simulink model "motor_kit_sim_20MHz"  (R2021b)
settings: Solver=VariableStepAuto  StartTime=0.0  StopTime=10*62.5E-6  RelTol=1e-3  EnableMultiTasking=on
PreLoadFcn:
  | setup_motor_kit_sim_20MHz;
InitFcn:
  | setup_motor_kit_sim_20MHz;
values from neighbouring files (symbols this model uses):
  DSPBASampleTime = 0.05e-6    (= 5e-08)    [setup_motor_kit_sim_20MHz.m]
  wordLength = 16    [setup_motor_kit_sim_20MHz.m]
undefined symbols (not defined in the file or in its folder): AdvDSPBChannelOutDisplay, dpoly, dspba_ChannelInVis, dspba_ChannelOutVis, dspba_internal_get_channel_ports, evalAionMaskParam, latency, primtype, value, x
libraries: DSPBAPrim x324, DSPBAModelBus x25, DSPBABase x7, dspsrcs4 x3, simulink x3, DSPBAUtilities x1
(part 4 of 5)

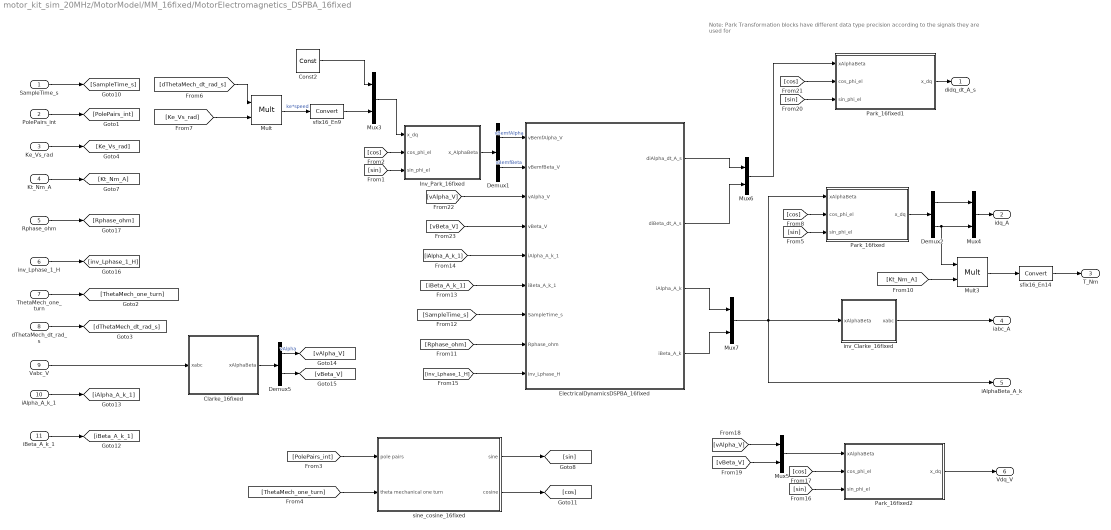
== system motor_kit_sim_20MHz/MotorModel/MM_16fixed/MotorElectromagnetics_DSPBA_16fixed ==
  note: Note: Park Transformation blocks have different data type precision according to the signals they are used for
  SampleTime_s : Inport
  PolePairs_int : Inport  Port=2
  Ke_Vs_rad : Inport  Port=3
  Kt_Nm_A : Inport  Port=4
  Rphase_ohm : Inport  Port=5
  inv_Lphase_1_H : Inport  Port=6
  ThetaMech_one_turn : Inport  Port=7
  dThetaMech_dt_rad_s : Inport  Port=8
  Vabc_V : Inport  Port=9
  iAlpha_A_k_1 : Inport  Port=10
  iBeta_A_k_1 : Inport  Port=11
  Clarke_16fixed : Subsystem
  Const2 : DSPBAPrim/Const  primtype=const  nInputs=0  nOutputs=1  omode=Specify via dialog  otype=DataType  scale=constScaleVoltage  rndmethod=Unbiased  factor=1  satmethod=Symmetric  shift_vec=[0 1 2 -1]  value=0  inPortNames=['+'; '+';]  outPortNames=[' ']  dspbaimage=dspba_prim.svg  text=fprintf('%s', num2str(value));  style=Optimised  visibilities=8 + 1024  floatPrecision=float32_m23  warnSaturation=on  version=20211007  SampleTime=inf
  Demux1 : Demux  Outputs=2
  Demux2 : Demux  Outputs=2
  Demux5 : Demux  Outputs=2
  ElectricalDynamicsDSPBA_16fixed : Subsystem
  Inv_Park_16fixed : Subsystem
  Mult : DSPBAPrim/Mult  primtype=mult  nInputs=2  nOutputs=1  omode=Inherit via internal rule  otype=DataType  scale=constScaleVoltage  rndmethod=Unbiased  factor=1  satmethod=Symmetric  shift_vec=[0 1 2 -1]  value=0  inPortNames=[' '; ' ';]  outPortNames=[' ']  dspbaimage=dspba_prim.svg  text=fprintf('X');  style=Optimised  visibilities=8+2^18+2^19  floatPrecision=float32_m23  floatRounding=correct  advOptions=[]  version=20211007
  Mult3 : DSPBAPrim/Mult  primtype=mult  nInputs=2  nOutputs=1  omode=Inherit via internal rule  otype=DataType  scale=constScaleTorque  rndmethod=Unbiased  factor=1  satmethod=Symmetric  shift_vec=[0 1 2 -1]  value=0  inPortNames=[' '; ' ';]  outPortNames=[' ']  dspbaimage=dspba_prim.svg  text=fprintf('X');  style=Optimised  visibilities=8+2^18+2^19  floatPrecision=float32_m23  floatRounding=correct  advOptions=[]  version=20211007
  Mux{3..7} (5 alike) : Mux  Inputs=2
  Park_16fixed : Subsystem
  Park_16fixed1 : Subsystem
  Park_16fixed2 : Subsystem
  inv_Clarke_16fixed : Subsystem
  sfix16_En14 : DSPBAPrim/Convert  primtype=convert  nInputs=1  nOutputs=1  omode=Specify via dialog  otype=DataTypeTorque  scale=constScaleTorque  rndmethod=Unbiased  factor=1  satmethod=Symmetric  shift_vec=[0 1 2 -1]  value=round([0:255]/17)  inPortNames=[' '; ' ';]  outPortNames=[' '; 'c']  dspbaimage=dspba_prim_wide.svg  text=fprintf('convert');  style=Optimised  visibilities=8+64+256+2^17  clipdetect=off  floatPrecision=float32_m23  advOptions=[]  version=20211007
  sfix16_En9 : DSPBAPrim/Convert  primtype=convert  nInputs=1  nOutputs=1  omode=Specify via dialog  otype=DataType  scale=constScaleVoltage  rndmethod=Unbiased  factor=1  satmethod=Symmetric  shift_vec=[0 1 2 -1]  value=round([0:255]/17)  inPortNames=[' '; ' ';]  outPortNames=[' '; 'c']  dspbaimage=dspba_prim_wide.svg  text=fprintf('convert');  style=Optimised  visibilities=8+64+256+2^17  clipdetect=off  floatPrecision=float32_m23  advOptions=[]  version=20211007
  sine_cosine_16fixed : Subsystem
  didq_dt_A_s : Outport
  idq_A : Outport  Port=2
  T_Nm : Outport  Port=3
  iabc_A : Outport  Port=4
  iAlphaBeta_A_k : Outport  Port=5
  Vdq_V : Outport  Port=6
  wires:
  Mult3/1 -> sfix16_En14/1
  [Kt_Nm_A] -> Mult3/2
  sine_cosine_16fixed/2(cosine) -> [cos]
  sine_cosine_16fixed/1(sine) -> [sin]
  [ThetaMech_one_turn] -> sine_cosine_16fixed/2(theta mechanical one turn)
  [PolePairs_int] -> sine_cosine_16fixed/1(pole pairs)
  Park_16fixed2/1(x_dq) -> Vdq_V/1
  [sin] -> Park_16fixed2/3(sin_phi_el)
  [cos] -> Park_16fixed2/2(cos_phi_el)
  Mux5/1 -> Park_16fixed2/1(xAlphaBeta)
  [vAlpha_V] -> Mux5/1
  [vBeta_V] -> Mux5/2
  inv_Clarke_16fixed/1(xabc) -> iabc_A/1
  Mux7/1 -> iAlphaBeta_A_k/1, Park_16fixed/1(xAlphaBeta), inv_Clarke_16fixed/1(xAlphaBeta)
  Mux4/1 -> idq_A/1
  Demux2/2 -> Mux4/2, Mult3/1
  Demux2/1 -> Mux4/1
  [sin] -> Park_16fixed/3(sin_phi_el)
  [cos] -> Park_16fixed/2(cos_phi_el)
  Park_16fixed/1(x_dq) -> Demux2/1
  Park_16fixed1/1(x_dq) -> didq_dt_A_s/1
  ElectricalDynamicsDSPBA_16fixed/2(diBeta_dt_A_s) -> Mux6/2
  ElectricalDynamicsDSPBA_16fixed/1(diAlpha_dt_A_s) -> Mux6/1
  [sin] -> Inv_Park_16fixed/3(sin_phi_el)
  [cos] -> Inv_Park_16fixed/2(cos_phi_el)
  [cos] -> Park_16fixed1/2(cos_phi_el)
  Mux6/1 -> Park_16fixed1/1(xAlphaBeta)
  [sin] -> Park_16fixed1/3(sin_phi_el)
  [inv_Lphase_1_H] -> ElectricalDynamicsDSPBA_16fixed/9(inv_Lphase_H)
  [Rphase_ohm] -> ElectricalDynamicsDSPBA_16fixed/8(Rphase_ohm)
  [SampleTime_s] -> ElectricalDynamicsDSPBA_16fixed/7(SampleTime_s)
  [iBeta_A_k_1] -> ElectricalDynamicsDSPBA_16fixed/6(iBeta_A_k_1)
  [iAlpha_A_k_1] -> ElectricalDynamicsDSPBA_16fixed/5(iAlpha_A_k_1)
  Mult/1 -> sfix16_En9/1  "ke*speed"
  [Ke_Vs_rad] -> Mult/2
  [dThetaMech_dt_rad_s] -> Mult/1
  Const2/1 -> Mux3/1
  iBeta_A_k_1/1 -> [iBeta_A_k_1]
  iAlpha_A_k_1/1 -> [iAlpha_A_k_1]
  dThetaMech_dt_rad_s/1 -> [dThetaMech_dt_rad_s]
  ThetaMech_one_turn/1 -> [ThetaMech_one_turn]
  inv_Lphase_1_H/1 -> [inv_Lphase_1_H]
  Rphase_ohm/1 -> [Rphase_ohm]
  Kt_Nm_A/1 -> [Kt_Nm_A]
  Ke_Vs_rad/1 -> [Ke_Vs_rad]
  SampleTime_s/1 -> [SampleTime_s]
  PolePairs_int/1 -> [PolePairs_int]
  Mux3/1 -> Inv_Park_16fixed/1(x_dq)
  Demux1/2 -> ElectricalDynamicsDSPBA_16fixed/2(vBemfBeta_V)  "vBemfBeta"
  Demux1/1 -> ElectricalDynamicsDSPBA_16fixed/1(vBemfAlpha_V)  "vBemfAlpha"
  Inv_Park_16fixed/1(x_AlphaBeta) -> Demux1/1
  [vAlpha_V] -> ElectricalDynamicsDSPBA_16fixed/3(vAlpha_V)
  [vBeta_V] -> ElectricalDynamicsDSPBA_16fixed/4(vBeta_V)
  Clarke_16fixed/1(xAlphaBeta) -> Demux5/1
  Demux5/2 -> [vBeta_V]
  Demux5/1 -> [vAlpha_V]  "vAlpha"
  Vabc_V/1 -> Clarke_16fixed/1(xabc)
  sfix16_En9/1 -> Mux3/2
  ElectricalDynamicsDSPBA_16fixed/4(iBeta_A_k) -> Mux7/2
  ElectricalDynamicsDSPBA_16fixed/3(iAlpha_A_k) -> Mux7/1
  sfix16_En14/1 -> T_Nm/1

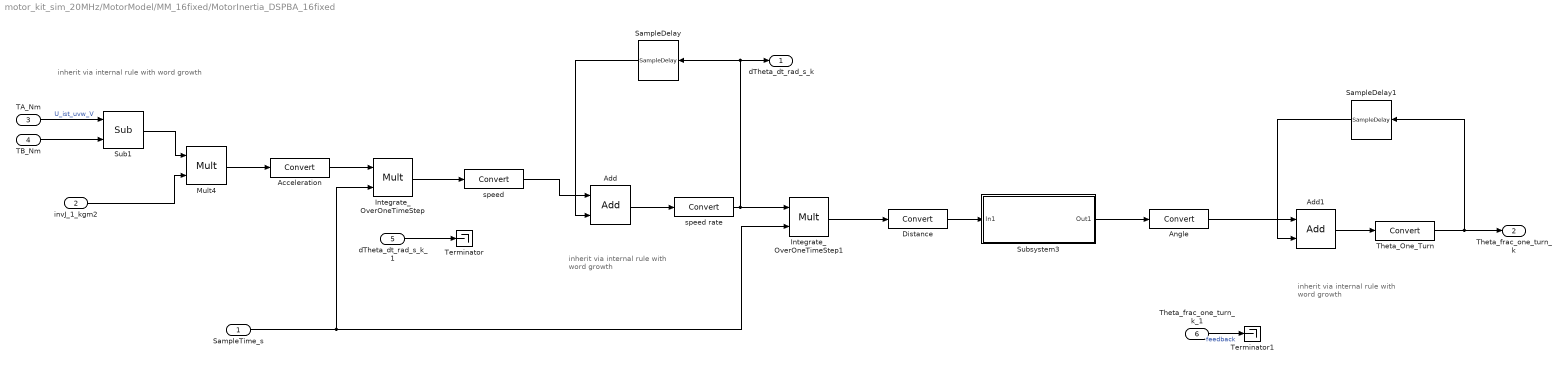
== system motor_kit_sim_20MHz/MotorModel/MM_16fixed/MotorInertia_DSPBA_16fixed ==
  note: inherit via internal rule with word growth
  note: inherit via internal rule
      | with word growth
  note: inherit via internal rule
      | with word growth
  SampleTime_s : Inport
  invJ_1_kgm2 : Inport  Port=2
  TA_Nm : Inport  Port=3
  TB_Nm : Inport  Port=4
  dTheta_dt_rad_s_k_1 : Inport  Port=5
  Theta_frac_one_turn_k_1 : Inport  Port=6
  Acceleration : DSPBAPrim/Convert  primtype=convert  nInputs=1  nOutputs=1  omode=Specify via dialog  otype=DataTypeAcceleration  scale=constScaleAcceleration  rndmethod=Truncate  factor=1  satmethod=None  shift_vec=[0 1 2 -1]  value=round([0:255]/17)  inPortNames=[' '; ' ';]  outPortNames=[' '; 'c']  dspbaimage=dspba_prim_wide.svg  text=fprintf('convert');  style=Optimised  visibilities=8+64+256+2^17  clipdetect=off  floatPrecision=float32_m23  advOptions=[]  version=20211007
  Add : DSPBAPrim/Add  primtype=add  nInputs=evalAionMaskParam(gcb,'value',1)  nOutputs=1  omode=Inherit via internal rule with word growth  otype=DataType  scale=constScaleSpeed  rndmethod=Unbiased  factor=1  satmethod=Symmetric  shift_vec=[0 1 2 -1]  value=2  inPortNames=[' '; ' ';]  outPortNames=[' ']  dspbaimage=dspba_prim.svg  text=fprintf('+');  style=Optimised  visibilities=1032  genFPC=off  floatRounding=correct  advOptions=[]  version=20211007
  Add1 : DSPBAPrim/Add  primtype=add  nInputs=evalAionMaskParam(gcb,'value',1)  nOutputs=1  omode=Inherit via internal rule with word growth  otype=DataTypeUnsigned  scale=2^-16  rndmethod=Unbiased  factor=1  satmethod=Symmetric  shift_vec=[0 1 2 -1]  value=2  inPortNames=[' '; ' ';]  outPortNames=[' ']  dspbaimage=dspba_prim.svg  text=fprintf('+');  style=Optimised  visibilities=1032  genFPC=off  floatRounding=correct  advOptions=[]  version=20211007
  Angle : DSPBAPrim/Convert  primtype=convert  nInputs=1  nOutputs=1  omode=Specify via dialog  otype=DataTypeTheta_OneTurn  scale=constScaleTheta_OneTurn  rndmethod=Unbiased  factor=1  satmethod=None  shift_vec=[0 1 2 -1]  value=round([0:255]/17)  inPortNames=[' '; ' ';]  outPortNames=[' '; 'c']  dspbaimage=dspba_prim_wide.svg  text=fprintf('convert');  style=Optimised  visibilities=8+64+256+2^17  clipdetect=off  floatPrecision=float32_m23  advOptions=[]  version=20211007
  Distance : DSPBAPrim/Convert  primtype=convert  nInputs=1  nOutputs=1  omode=Specify via dialog  otype=DataTypeDis  scale=constScaleDis  rndmethod=Unbiased  factor=1  satmethod=None  shift_vec=[0 1 2 -1]  value=round([0:255]/17)  inPortNames=[' '; ' ';]  outPortNames=[' '; 'c']  dspbaimage=dspba_prim_wide.svg  text=fprintf('convert');  style=Optimised  visibilities=8+64+256+2^17  clipdetect=off  floatPrecision=float32_m23  advOptions=[]  version=20211007
  Integrate_OverOneTimeStep : DSPBAPrim/Mult  primtype=mult  nInputs=2  nOutputs=1  omode=Inherit via internal rule  otype=DataType  scale=2^-12  rndmethod=Unbiased  factor=1  satmethod=Symmetric  shift_vec=[0 1 2 -1]  value=0  inPortNames=[' '; ' ';]  outPortNames=[' ']  dspbaimage=dspba_prim.svg  text=fprintf('X');  style=Optimised  visibilities=8+2^18+2^19  floatPrecision=float32_m23  floatRounding=correct  advOptions=[]  version=20211007
  Integrate_OverOneTimeStep1 : DSPBAPrim/Mult  primtype=mult  nInputs=2  nOutputs=1  omode=Inherit via internal rule  otype=sfix(32)  scale=2^-28  rndmethod=Unbiased  factor=1  satmethod=Symmetric  shift_vec=[0 1 2 -1]  value=0  inPortNames=[' '; ' ';]  outPortNames=[' ']  dspbaimage=dspba_prim.svg  text=fprintf('X');  style=Optimised  visibilities=8+2^18+2^19  floatPrecision=float32_m23  floatRounding=correct  advOptions=[]  version=20211007
  Mult4 : DSPBAPrim/Mult  primtype=mult  nInputs=2  nOutputs=1  omode=Inherit via internal rule  otype=DataTypeAcceleration  scale=2^0  rndmethod=Unbiased  factor=1  satmethod=Symmetric  shift_vec=[0 1 2 -1]  value=0  inPortNames=[' '; ' ';]  outPortNames=[' ']  dspbaimage=dspba_prim.svg  text=fprintf('X');  style=Optimised  visibilities=8+2^18+2^19  floatPrecision=float32_m23  floatRounding=correct  advOptions=[]  version=20211007
  SampleDelay : DSPBAPrim/SampleDelay  primtype=sampdelay  nInputs=1  nOutputs=1  omode=Inherit via internal rule  otype=sfix(16)  scale=2^-15  rndmethod=Unbiased  factor=1  satmethod=Symmetric  shift_vec=[0 1 2 -1]  floatPrecision=float32_m23  value=1  inPortNames=[' '; ' ';]  outPortNames=[' ']  dspbaimage=dspba_prim.svg  text=dpoly(1, eye(1,value+1), 'z')  style=Optimised  visibilities=8 + 1024 + 2^17 + 2^18  flexible=off  slackgroup=0  augmented=0  version=20211007  advOptions=[]
  SampleDelay1 : DSPBAPrim/SampleDelay  primtype=sampdelay  nInputs=1  nOutputs=1  omode=Inherit via internal rule  otype=sfix(16)  scale=2^-15  rndmethod=Unbiased  factor=1  satmethod=Symmetric  shift_vec=[0 1 2 -1]  floatPrecision=float32_m23  value=1  inPortNames=[' '; ' ';]  outPortNames=[' ']  dspbaimage=dspba_prim.svg  text=dpoly(1, eye(1,value+1), 'z')  style=Optimised  visibilities=8 + 1024 + 2^17 + 2^18  flexible=off  slackgroup=0  augmented=0  version=20211007  advOptions=[]
  Sub1 : DSPBAPrim/Sub  primtype=sub  nInputs=2  nOutputs=1  omode=Inherit via internal rule with word growth  otype=DataType  scale=constScaleTorque  rndmethod=Unbiased  factor=1  satmethod=Symmetric  shift_vec=[0 1 2 -1]  value=0  inPortNames=['+'; '-';]  outPortNames=[' ']  dspbaimage=dspba_prim.svg  text=fprintf('-');  style=Optimised  visibilities=8+2^17+2^18  floatRounding=correct  advOptions=[]  version=20211007
  Subsystem3 : Subsystem  mask{constVal=1/(2*pi)}
      mask prompts: constVal "Scaling phi elec"
      mask Display:
      | color('w');
      | set_param(gcb,'BackgroundColor','yellow');
      | fprintf('Scaling phi mech\n%s', num2str(constVal));
      | port_label('input',1, 'rad');
      | port_label('output',1,'turns');
  Terminator : Terminator
  Terminator1 : Terminator
  Theta_One_Turn : DSPBAPrim/Convert  primtype=convert  nInputs=1  nOutputs=1  omode=Specify via dialog  otype=DataTypeTheta_OneTurn  scale=constScaleTheta_OneTurn  rndmethod=Unbiased  factor=1  satmethod=None  shift_vec=[0 1 2 -1]  value=round([0:255]/17)  inPortNames=[' '; ' ';]  outPortNames=[' '; 'c']  dspbaimage=dspba_prim_wide.svg  text=fprintf('convert');  style=Optimised  visibilities=8+64+256+2^17  clipdetect=off  floatPrecision=float32_m23  advOptions=[]  version=20211007
  speed : DSPBAPrim/Convert  primtype=convert  nInputs=1  nOutputs=1  omode=Specify via dialog  otype=DataTypeSpeed  scale=constScaleSpeed  rndmethod=Unbiased  factor=1  satmethod=None  shift_vec=[0 1 2 -1]  value=round([0:255]/17)  inPortNames=[' '; ' ';]  outPortNames=[' '; 'c']  dspbaimage=dspba_prim_wide.svg  text=fprintf('convert');  style=Optimised  visibilities=8+64+256+2^17  clipdetect=off  floatPrecision=float32_m23  advOptions=[]  version=20211007
  speed rate : DSPBAPrim/Convert  primtype=convert  nInputs=1  nOutputs=1  omode=Specify via dialog  otype=DataTypeSpeedRate  scale=constScaleSpeedRate  rndmethod=Unbiased  factor=1  satmethod=None  shift_vec=[0 1 2 -1]  value=round([0:255]/17)  inPortNames=[' '; ' ';]  outPortNames=[' '; 'c']  dspbaimage=dspba_prim_wide.svg  text=fprintf('convert');  style=Optimised  visibilities=8+64+256+2^17  clipdetect=off  floatPrecision=float32_m23  advOptions=[]  version=20211007
  dTheta_dt_rad_s_k : Outport
  Theta_frac_one_turn_k : Outport  Port=2
  wires:
  Sub1/1 -> Mult4/1
  Add1/1 -> Theta_One_Turn/1
  Subsystem3/1(Out1) -> Angle/1
  SampleTime_s/1 -> Integrate_OverOneTimeStep/2, Integrate_OverOneTimeStep1/2
  TB_Nm/1 -> Sub1/2
  TA_Nm/1 -> Sub1/1  "U_ist_uvw_V"
  invJ_1_kgm2/1 -> Mult4/2
  Add/1 -> speed rate/1
  Integrate_OverOneTimeStep/1 -> speed/1
  Mult4/1 -> Acceleration/1
  Acceleration/1 -> Integrate_OverOneTimeStep/1
  speed/1 -> Add/1
  speed rate/1 -> dTheta_dt_rad_s_k/1, SampleDelay/1, Integrate_OverOneTimeStep1/1
  Distance/1 -> Subsystem3/1(In1)
  Integrate_OverOneTimeStep1/1 -> Distance/1
  Angle/1 -> Add1/1
  Theta_One_Turn/1 -> SampleDelay1/1, Theta_frac_one_turn_k/1
  SampleDelay/1 -> Add/2
  dTheta_dt_rad_s_k_1/1 -> Terminator/1
  SampleDelay1/1 -> Add1/2
  Theta_frac_one_turn_k_1/1 -> Terminator1/1  "feedback"

== system motor_kit_sim_20MHz/MotorModel/MM_16fixed/inverter ==
  note: If high transistor is connected, current is drawn from DC link.
      | Total DC link current is sum of currents flowing from DC link to motor terminals.
  note: Three motor terminal voltages.
  dc_link_V : Inport
  uvw_h : Inport  Port=2  OutDataTypeStr=boolean
  uvw_l : Inport  Port=3  OutDataTypeStr=boolean
  Iabc_A : Inport  Port=4
  Add3 : DSPBAPrim/Add  primtype=add  nInputs=evalAionMaskParam(gcb,'value',1)  nOutputs=1  omode=Specify via dialog  otype=sfix(19)  scale=2^-10  rndmethod=Unbiased  factor=1  satmethod=Symmetric  shift_vec=[0 1 2 -1]  value=3  inPortNames=[' '; ' ';]  outPortNames=[' ']  dspbaimage=dspba_prim.svg  text=fprintf('+');  style=Optimised  visibilities=1032+2^17+2^18+2^19  genFPC=off  floatRounding=correct  advOptions=[]  version=20211007
  Demux1 : Demux  Outputs=3
  Demux4 : Demux  Outputs=3
  Mult{,1..3} (4 alike) : DSPBAPrim/Mult  primtype=mult  nInputs=2  nOutputs=1  omode=Inherit via internal rule  otype=DataType  scale=constScaleVoltage  rndmethod=Unbiased  factor=1  satmethod=Symmetric  shift_vec=[0 1 2 -1]  value=0  inPortNames=[' '; ' ';]  outPortNames=[' ']  dspbaimage=dspba_prim.svg  text=fprintf('X');  style=Optimised  visibilities=8+2^18+2^19  floatPrecision=float32_m23  floatRounding=correct  advOptions=[]  version=20211007
  Terminator4 : Terminator
  Vabc_V : Outport
  dc_link_current_A : Outport  Port=2
  wires:
  Mult/1 -> Vabc_V/1
  dc_link_V/1 -> Mult/1
  uvw_h/1 -> Demux4/1, Mult/2
  uvw_l/1 -> Terminator4/1
  Iabc_A/1 -> Demux1/1
  Demux4/1 -> Mult1/1
  Demux1/1 -> Mult1/2
  Demux4/2 -> Mult2/1
  Demux1/2 -> Mult2/2
  Demux4/3 -> Mult3/1
  Demux1/3 -> Mult3/2
  Mult1/1 -> Add3/1
  Mult2/1 -> Add3/2
  Mult3/1 -> Add3/3
  Add3/1 -> dc_link_current_A/1

== system motor_kit_sim_20MHz/MotorModel/MM_16fixed/MotorElectromagnetics_DSPBA_16fixed/Clarke_16fixed ==
  note: or:
      | (xb+xc) * (-0.5) + xa
  note: Transformation from 3-phase stator coil values to equivalent 2-phase values.
      | Scaling chosen so peak values remain the same.
      | Transformation equations:
      |
      | xAlpha = 2/3*(xa - 0.5*xb - 0.5*xc)
      | xBeta = 2/3*(sqrt(3)/2*xb - sqrt(3)/2*xc)
  xabc : Inport
  Add1 : DSPBAPrim/Add  primtype=add  nInputs=evalAionMaskParam(gcb,'value',1)  nOutputs=1  omode=Inherit via internal rule with word growth  otype=sfix(17)  scale=constScaleVoltage  rndmethod=Unbiased  factor=1  satmethod=Symmetric  shift_vec=[0 1 2 -1]  value=3  inPortNames=[' '; ' ';]  outPortNames=[' ']  dspbaimage=dspba_prim.svg  text=fprintf('+');  style=Optimised  visibilities=1032+2^17+2^18+2^19  genFPC=off  floatRounding=correct  advOptions=[]  version=20211007
  Demux1 : Demux  Outputs=2
  Demux2 : Demux  Outputs=2
  Demux4 : Demux  Outputs=3
  Mux1 : Mux  Inputs=2
  Mux2 : Mux  Inputs=2
  Sub1 : DSPBAPrim/Sub  primtype=sub  nInputs=2  nOutputs=1  omode=Inherit via internal rule with word growth  otype=sfix(17)  scale=constScaleVoltage  rndmethod=Unbiased  factor=1  satmethod=Symmetric  shift_vec=[0 1 2 -1]  value=0  inPortNames=['+'; '-';]  outPortNames=[' ']  dspbaimage=dspba_prim.svg  text=fprintf('-');  style=Optimised  visibilities=8+2^17+2^18  floatRounding=correct  advOptions=[]  version=20211007
  Subsystem1 : Subsystem  mask{constVal=2/3}
      mask prompts: constVal "Gain"
      mask Display:
      | color('w');
      | set_param(gcb,'BackgroundColor','yellow');
      | fprintf('Gain\n%s', num2str(constVal));
      | port_label('input',1, 'a');
      | port_label('output',1,'b');
  Subsystem2 : Subsystem  mask{constVal=sqrt(3)/2}
      mask prompts: constVal "Gain"
      mask Display:
      | color('w');
      | set_param(gcb,'BackgroundColor','yellow');
      | fprintf('Gain\n%s', num2str(constVal));
      | port_label('input',1, 'a');
      | port_label('output',1,'b');
  Subsystem6 : Subsystem  mask{constVal=-1/2}
      mask prompts: constVal "Gain"
      mask Display:
      | color('w');
      | set_param(gcb,'BackgroundColor','yellow');
      | fprintf('Gain\n%s', num2str(constVal));
      | port_label('input',1, 'a');
      | port_label('output',1,'b');
  sfix16_En9_1 : DSPBAPrim/Convert  primtype=convert  nInputs=1  nOutputs=1  omode=Specify via dialog  otype=DataType  scale=constScaleVoltage  rndmethod=Unbiased  factor=1  satmethod=Symmetric  shift_vec=[0 1 2 -1]  value=round([0:255]/17)  inPortNames=[' '; ' ';]  outPortNames=[' '; 'c']  dspbaimage=dspba_prim_wide.svg  text=fprintf('convert');  style=Optimised  visibilities=8+64+256+2^17  clipdetect=off  floatPrecision=float32_m23  advOptions=[]  version=20211007
  sfix16_En9_2 : DSPBAPrim/Convert  primtype=convert  nInputs=1  nOutputs=1  omode=Specify via dialog  otype=DataType  scale=constScaleVoltage  rndmethod=Unbiased  factor=1  satmethod=Symmetric  shift_vec=[0 1 2 -1]  value=round([0:255]/17)  inPortNames=[' '; ' ';]  outPortNames=[' '; 'c']  dspbaimage=dspba_prim_wide.svg  text=fprintf('convert');  style=Optimised  visibilities=8+64+256+2^17  clipdetect=off  floatPrecision=float32_m23  advOptions=[]  version=20211007
  sfix16_En9_3 : DSPBAPrim/Convert  primtype=convert  nInputs=1  nOutputs=1  omode=Specify via dialog  otype=DataType  scale=constScaleVoltage  rndmethod=Unbiased  factor=1  satmethod=Symmetric  shift_vec=[0 1 2 -1]  value=round([0:255]/17)  inPortNames=[' '; ' ';]  outPortNames=[' '; 'c']  dspbaimage=dspba_prim_wide.svg  text=fprintf('convert');  style=Optimised  visibilities=8+64+256+2^17  clipdetect=off  floatPrecision=float32_m23  advOptions=[]  version=20211007
  xAlphaBeta : Outport
  wires:
  xabc/1 -> Demux4/1
  Demux4/2 -> Mux1/1  "xb"
  Demux4/3 -> Mux1/2  "xc"
  Mux1/1 -> Subsystem2/1(In1), Subsystem6/1(In1)
  Subsystem6/1(Out1) -> Demux1/1
  Demux4/1 -> Add1/1  "xa"
  Demux1/1 -> Add1/2  "-0.5*xb"
  Demux1/2 -> Add1/3  "-0.5*xc"
  Subsystem2/1(Out1) -> Demux2/1
  Demux2/1 -> Sub1/1  "(sqrt(3)/2)*xb"
  Demux2/2 -> Sub1/2  "(sqrt(3)/2)*xc"
  Mux2/1 -> Subsystem1/1(In1)
  Add1/1 -> sfix16_En9_2/1
  Sub1/1 -> sfix16_En9_1/1
  Subsystem1/1(Out1) -> sfix16_En9_3/1
  sfix16_En9_1/1 -> Mux2/2
  sfix16_En9_2/1 -> Mux2/1
  sfix16_En9_3/1 -> xAlphaBeta/1

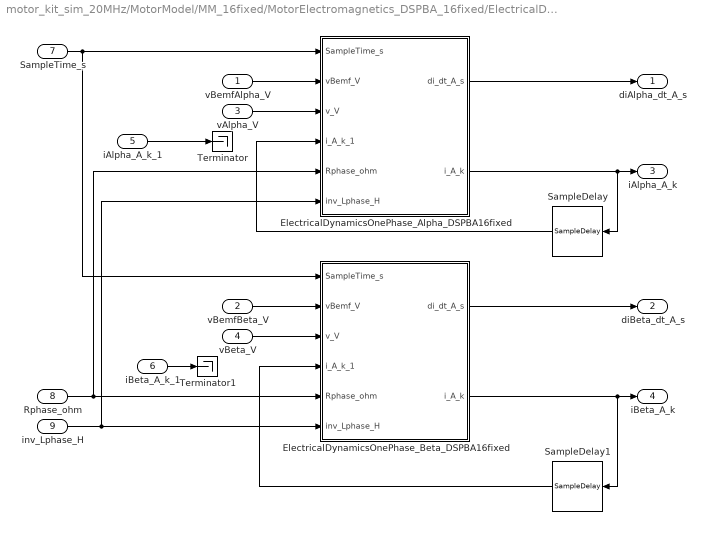
== system motor_kit_sim_20MHz/MotorModel/MM_16fixed/MotorElectromagnetics_DSPBA_16fixed/ElectricalDynamicsDSPBA_16fixed ==
  vBemfAlpha_V : Inport
  vBemfBeta_V : Inport  Port=2
  vAlpha_V : Inport  Port=3
  vBeta_V : Inport  Port=4
  iAlpha_A_k_1 : Inport  Port=5
  iBeta_A_k_1 : Inport  Port=6
  SampleTime_s : Inport  Port=7
  Rphase_ohm : Inport  Port=8
  inv_Lphase_H : Inport  Port=9
  ElectricalDynamicsOnePhase_Alpha_DSPBA16fixed : Subsystem
  ElectricalDynamicsOnePhase_Beta_DSPBA16fixed : Subsystem
  SampleDelay : DSPBAPrim/SampleDelay  primtype=sampdelay  nInputs=1  nOutputs=1  omode=Inherit via internal rule  otype=sfix(16)  scale=2^-15  rndmethod=Unbiased  factor=1  satmethod=Symmetric  shift_vec=[0 1 2 -1]  floatPrecision=float32_m23  value=20  inPortNames=[' '; ' ';]  outPortNames=[' ']  dspbaimage=dspba_prim.svg  text=dpoly(1, eye(1,value+1), 'z')  style=Optimised  visibilities=8 + 1024 + 2^17 + 2^18  flexible=off  slackgroup=0  augmented=0  version=20211007  advOptions=[]
  SampleDelay1 : DSPBAPrim/SampleDelay  primtype=sampdelay  nInputs=1  nOutputs=1  omode=Inherit via internal rule  otype=sfix(16)  scale=2^-15  rndmethod=Unbiased  factor=1  satmethod=Symmetric  shift_vec=[0 1 2 -1]  floatPrecision=float32_m23  value=20  inPortNames=[' '; ' ';]  outPortNames=[' ']  dspbaimage=dspba_prim.svg  text=dpoly(1, eye(1,value+1), 'z')  style=Optimised  visibilities=8 + 1024 + 2^17 + 2^18  flexible=off  slackgroup=0  augmented=0  version=20211007  advOptions=[]
  Terminator : Terminator
  Terminator1 : Terminator
  diAlpha_dt_A_s : Outport
  diBeta_dt_A_s : Outport  Port=2
  iAlpha_A_k : Outport  Port=3
  iBeta_A_k : Outport  Port=4
  wires:
  vBeta_V/1 -> ElectricalDynamicsOnePhase_Beta_DSPBA16fixed/3(v_V)
  ElectricalDynamicsOnePhase_Beta_DSPBA16fixed/1(di_dt_A_s) -> diBeta_dt_A_s/1
  vBemfBeta_V/1 -> ElectricalDynamicsOnePhase_Beta_DSPBA16fixed/2(vBemf_V)
  SampleTime_s/1 -> ElectricalDynamicsOnePhase_Alpha_DSPBA16fixed/1(SampleTime_s), ElectricalDynamicsOnePhase_Beta_DSPBA16fixed/1(SampleTime_s)
  ElectricalDynamicsOnePhase_Alpha_DSPBA16fixed/2(i_A_k) -> SampleDelay/1, iAlpha_A_k/1
  ElectricalDynamicsOnePhase_Alpha_DSPBA16fixed/1(di_dt_A_s) -> diAlpha_dt_A_s/1
  Rphase_ohm/1 -> ElectricalDynamicsOnePhase_Beta_DSPBA16fixed/5(Rphase_ohm), ElectricalDynamicsOnePhase_Alpha_DSPBA16fixed/5(Rphase_ohm)
  inv_Lphase_H/1 -> ElectricalDynamicsOnePhase_Beta_DSPBA16fixed/6(inv_Lphase_H), ElectricalDynamicsOnePhase_Alpha_DSPBA16fixed/6(inv_Lphase_H)
  vAlpha_V/1 -> ElectricalDynamicsOnePhase_Alpha_DSPBA16fixed/3(v_V)
  vBemfAlpha_V/1 -> ElectricalDynamicsOnePhase_Alpha_DSPBA16fixed/2(vBemf_V)
  ElectricalDynamicsOnePhase_Beta_DSPBA16fixed/2(i_A_k) -> SampleDelay1/1, iBeta_A_k/1
  SampleDelay/1 -> ElectricalDynamicsOnePhase_Alpha_DSPBA16fixed/4(i_A_k_1)
  iAlpha_A_k_1/1 -> Terminator/1
  iBeta_A_k_1/1 -> Terminator1/1
  SampleDelay1/1 -> ElectricalDynamicsOnePhase_Beta_DSPBA16fixed/4(i_A_k_1)

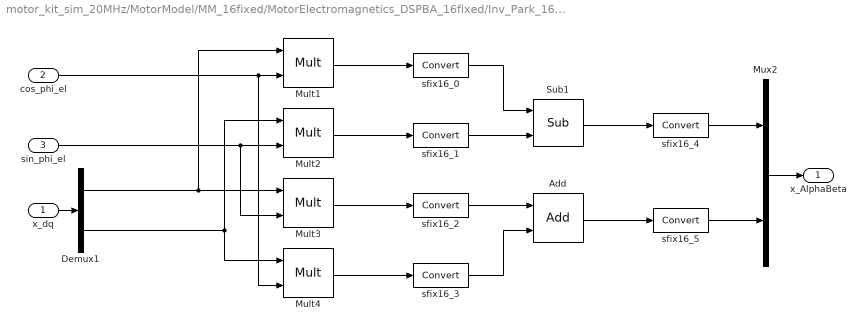
== system motor_kit_sim_20MHz/MotorModel/MM_16fixed/MotorElectromagnetics_DSPBA_16fixed/Inv_Park_16fixed ==
  x_dq : Inport
  cos_phi_el : Inport  Port=2
  sin_phi_el : Inport  Port=3
  Add : DSPBAPrim/Add  primtype=add  nInputs=evalAionMaskParam(gcb,'value',1)  nOutputs=1  omode=Inherit via internal rule with word growth  otype=sfix(17)  scale=constScaleVoltage  rndmethod=Unbiased  factor=1  satmethod=Symmetric  shift_vec=[0 1 2 -1]  value=2  inPortNames=[' '; ' ';]  outPortNames=[' ']  dspbaimage=dspba_prim.svg  text=fprintf('+');  style=Optimised  visibilities=1032  genFPC=off  floatRounding=correct  advOptions=[]  version=20211007
  Demux1 : Demux  Outputs=2
  Mult{1..4} (4 alike) : DSPBAPrim/Mult  primtype=mult  nInputs=2  nOutputs=1  omode=Inherit via internal rule  otype=DataType  scale=constScaleVoltage  rndmethod=Unbiased  factor=1  satmethod=Symmetric  shift_vec=[0 1 2 -1]  value=0  inPortNames=[' '; ' ';]  outPortNames=[' ']  dspbaimage=dspba_prim.svg  text=fprintf('X');  style=Optimised  visibilities=8+2^18+2^19  floatPrecision=float32_m23  floatRounding=correct  advOptions=[]  version=20211007
  Mux2 : Mux  Inputs=2
  Sub1 : DSPBAPrim/Sub  primtype=sub  nInputs=2  nOutputs=1  omode=Inherit via internal rule with word growth  otype=sfix(17)  scale=constScaleVoltage  rndmethod=Unbiased  factor=1  satmethod=Symmetric  shift_vec=[0 1 2 -1]  value=0  inPortNames=['+'; '-';]  outPortNames=[' ']  dspbaimage=dspba_prim.svg  text=fprintf('-');  style=Optimised  visibilities=8  floatRounding=correct  advOptions=[]  version=20211007
  sfix16_{0..5} (6 alike) : DSPBAPrim/Convert  primtype=convert  nInputs=1  nOutputs=1  omode=Specify via dialog  otype=DataType  scale=constScaleVoltage  rndmethod=Unbiased  factor=1  satmethod=Symmetric  shift_vec=[0 1 2 -1]  value=round([0:255]/17)  inPortNames=[' '; ' ';]  outPortNames=[' '; 'c']  dspbaimage=dspba_prim_wide.svg  text=fprintf('convert');  style=Optimised  visibilities=8+64+256+2^17  clipdetect=off  floatPrecision=float32_m23  advOptions=[]  version=20211007
  x_AlphaBeta : Outport
  wires:
  sin_phi_el/1 -> Mult2/2, Mult3/2
  Mult4/1 -> sfix16_3/1
  Mult3/1 -> sfix16_2/1
  Mult2/1 -> sfix16_1/1
  Mult1/1 -> sfix16_0/1
  Add/1 -> sfix16_5/1
  Sub1/1 -> sfix16_4/1
  Demux1/2 -> Mult2/1, Mult4/1
  Demux1/1 -> Mult1/1, Mult3/1
  x_dq/1 -> Demux1/1
  cos_phi_el/1 -> Mult1/2, Mult4/2
  Mux2/1 -> x_AlphaBeta/1
  sfix16_0/1 -> Sub1/1
  sfix16_1/1 -> Sub1/2
  sfix16_2/1 -> Add/1
  sfix16_3/1 -> Add/2
  sfix16_4/1 -> Mux2/1
  sfix16_5/1 -> Mux2/2

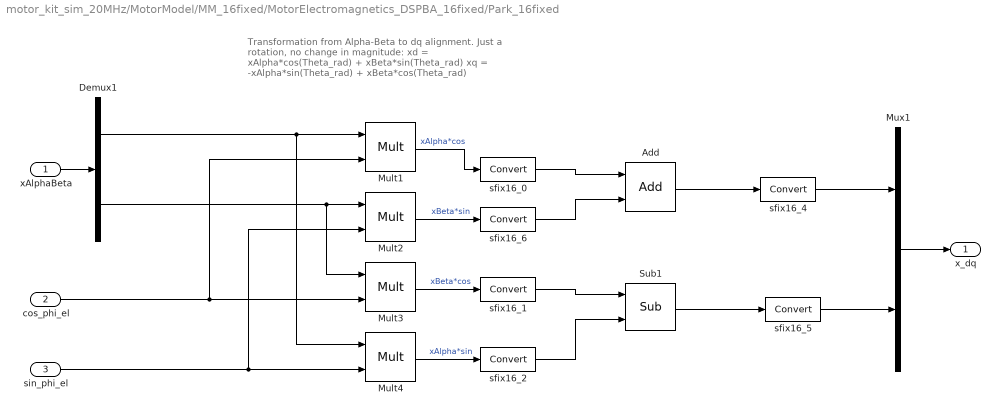
== system motor_kit_sim_20MHz/MotorModel/MM_16fixed/MotorElectromagnetics_DSPBA_16fixed/Park_16fixed ==
  note: Transformation from Alpha-Beta to dq alignment.
      | Just a rotation, no change in magnitude:
      |
      | xd = xAlpha*cos(Theta_rad) + xBeta*sin(Theta_rad)
      | xq = -xAlpha*sin(Theta_rad) + xBeta*cos(Theta_rad)
  xAlphaBeta : Inport
  cos_phi_el : Inport  Port=2
  sin_phi_el : Inport  Port=3
  Add : DSPBAPrim/Add  primtype=add  nInputs=evalAionMaskParam(gcb,'value',1)  nOutputs=1  omode=Inherit via internal rule with word growth  otype=sfix(17)  scale=constScaleCurrent  rndmethod=Unbiased  factor=1  satmethod=Symmetric  shift_vec=[0 1 2 -1]  value=2  inPortNames=[' '; ' ';]  outPortNames=[' ']  dspbaimage=dspba_prim.svg  text=fprintf('+');  style=Optimised  visibilities=1032  genFPC=off  floatRounding=correct  advOptions=[]  version=20211007
  Demux1 : Demux  Outputs=2
  Mult{1..4} (4 alike) : DSPBAPrim/Mult  primtype=mult  nInputs=2  nOutputs=1  omode=Inherit via internal rule  otype=DataType  scale=constScaleCurrent  rndmethod=Unbiased  factor=1  satmethod=Symmetric  shift_vec=[0 1 2 -1]  value=0  inPortNames=[' '; ' ';]  outPortNames=[' ']  dspbaimage=dspba_prim.svg  text=fprintf('X');  style=Optimised  visibilities=8+2^18+2^19  floatPrecision=float32_m23  floatRounding=correct  advOptions=[]  version=20211007
  Mux1 : Mux  Inputs=2
  Sub1 : DSPBAPrim/Sub  primtype=sub  nInputs=2  nOutputs=1  omode=Inherit via internal rule with word growth  otype=sfix(17)  scale=constScaleCurrent  rndmethod=Unbiased  factor=1  satmethod=Symmetric  shift_vec=[0 1 2 -1]  value=0  inPortNames=['+'; '-';]  outPortNames=[' ']  dspbaimage=dspba_prim.svg  text=fprintf('-');  style=Optimised  visibilities=8  floatRounding=correct  advOptions=[]  version=20211007
  sfix16_{0..2,6} (4 alike) : DSPBAPrim/Convert  primtype=convert  nInputs=1  nOutputs=1  omode=Specify via dialog  otype=sfix(43)  scale=2^-33  rndmethod=Unbiased  factor=1  satmethod=Symmetric  shift_vec=[0 1 2 -1]  value=round([0:255]/17)  inPortNames=[' '; ' ';]  outPortNames=[' '; 'c']  dspbaimage=dspba_prim_wide.svg  text=fprintf('convert');  style=Optimised  visibilities=8+64+256+2^17  clipdetect=off  floatPrecision=float32_m23  advOptions=[]  version=20211007
  sfix16_4 : DSPBAPrim/Convert  primtype=convert  nInputs=1  nOutputs=1  omode=Specify via dialog  otype=DataType_dq  scale=constScale_dq  rndmethod=Unbiased  factor=1  satmethod=Symmetric  shift_vec=[0 1 2 -1]  value=round([0:255]/17)  inPortNames=[' '; ' ';]  outPortNames=[' '; 'c']  dspbaimage=dspba_prim_wide.svg  text=fprintf('convert');  style=Optimised  visibilities=8+64+256+2^17  clipdetect=off  floatPrecision=float32_m23  advOptions=[]  version=20211007
  sfix16_5 : DSPBAPrim/Convert  primtype=convert  nInputs=1  nOutputs=1  omode=Specify via dialog  otype=DataType_dq  scale=constScale_dq  rndmethod=Unbiased  factor=1  satmethod=Symmetric  shift_vec=[0 1 2 -1]  value=round([0:255]/17)  inPortNames=[' '; ' ';]  outPortNames=[' '; 'c']  dspbaimage=dspba_prim_wide.svg  text=fprintf('convert');  style=Optimised  visibilities=8+64+256+2^17  clipdetect=off  floatPrecision=float32_m23  advOptions=[]  version=20211007
  x_dq : Outport
  wires:
  cos_phi_el/1 -> Mult3/2, Mult1/2
  Demux1/2 -> Mult3/1, Mult2/1
  sin_phi_el/1 -> Mult4/2, Mult2/2
  Mux1/1 -> x_dq/1
  Mult1/1 -> sfix16_0/1  "xAlpha*cos"
  Mult2/1 -> sfix16_6/1  "xBeta*sin"
  Demux1/1 -> Mult4/1, Mult1/1
  Mult4/1 -> sfix16_2/1  "xAlpha*sin"
  Mult3/1 -> sfix16_1/1  "xBeta*cos"
  xAlphaBeta/1 -> Demux1/1
  sfix16_0/1 -> Add/1
  sfix16_6/1 -> Add/2
  sfix16_1/1 -> Sub1/1
  sfix16_2/1 -> Sub1/2
  Sub1/1 -> sfix16_5/1
  Add/1 -> sfix16_4/1
  sfix16_4/1 -> Mux1/1
  sfix16_5/1 -> Mux1/2

== system motor_kit_sim_20MHz/MotorModel/MM_16fixed/MotorElectromagnetics_DSPBA_16fixed/Park_16fixed1 ==
  note: Transformation from Alpha-Beta to dq alignment.
      | Just a rotation, no change in magnitude:
      |
      | xd = xAlpha*cos(Theta_rad) + xBeta*sin(Theta_rad)
      | xq = -xAlpha*sin(Theta_rad) + xBeta*cos(Theta_rad)
  xAlphaBeta : Inport
  cos_phi_el : Inport  Port=2
  sin_phi_el : Inport  Port=3
  Add : DSPBAPrim/Add  primtype=add  nInputs=evalAionMaskParam(gcb,'value',1)  nOutputs=1  omode=Inherit via internal rule with word growth  otype=sfix(17)  scale=constScaleCurrentDerivative  rndmethod=Unbiased  factor=1  satmethod=Symmetric  shift_vec=[0 1 2 -1]  value=2  inPortNames=[' '; ' ';]  outPortNames=[' ']  dspbaimage=dspba_prim.svg  text=fprintf('+');  style=Optimised  visibilities=1032  genFPC=off  floatRounding=correct  advOptions=[]  version=20211007
  Demux1 : Demux  Outputs=2
  Mult{1..4} (4 alike) : DSPBAPrim/Mult  primtype=mult  nInputs=2  nOutputs=1  omode=Inherit via internal rule  otype=DataType  scale=constScaleCurrentDerivative  rndmethod=Unbiased  factor=1  satmethod=Symmetric  shift_vec=[0 1 2 -1]  value=0  inPortNames=[' '; ' ';]  outPortNames=[' ']  dspbaimage=dspba_prim.svg  text=fprintf('X');  style=Optimised  visibilities=8+2^18+2^19  floatPrecision=float32_m23  floatRounding=correct  advOptions=[]  version=20211007
  Mux1 : Mux  Inputs=2
  Sub1 : DSPBAPrim/Sub  primtype=sub  nInputs=2  nOutputs=1  omode=Inherit via internal rule with word growth  otype=sfix(17)  scale=constScaleCurrentDerivative  rndmethod=Unbiased  factor=1  satmethod=Symmetric  shift_vec=[0 1 2 -1]  value=0  inPortNames=['+'; '-';]  outPortNames=[' ']  dspbaimage=dspba_prim.svg  text=fprintf('-');  style=Optimised  visibilities=8  floatRounding=correct  advOptions=[]  version=20211007
  sfix16_En{1..4} (4 alike) : DSPBAPrim/Convert  primtype=convert  nInputs=1  nOutputs=1  omode=Specify via dialog  otype=sfix(32)  scale=2^-15  rndmethod=Unbiased  factor=1  satmethod=Symmetric  shift_vec=[0 1 2 -1]  value=round([0:255]/17)  inPortNames=[' '; ' ';]  outPortNames=[' '; 'c']  dspbaimage=dspba_prim_wide.svg  text=fprintf('convert');  style=Optimised  visibilities=8+64+256+2^17  clipdetect=off  floatPrecision=float32_m23  advOptions=[]  version=20211007
  x_dq : Outport
  wires:
  cos_phi_el/1 -> Mult3/2, Mult1/2
  Demux1/2 -> Mult3/1, Mult2/1
  sin_phi_el/1 -> Mult4/2, Mult2/2
  Mux1/1 -> x_dq/1
  Mult1/1 -> sfix16_En3/1
  Mult2/1 -> sfix16_En1/1
  Demux1/1 -> Mult4/1, Mult1/1
  Mult4/1 -> sfix16_En4/1
  Mult3/1 -> sfix16_En2/1
  xAlphaBeta/1 -> Demux1/1
  Add/1 -> Mux1/1
  Sub1/1 -> Mux1/2
  sfix16_En3/1 -> Add/1
  sfix16_En1/1 -> Add/2
  sfix16_En2/1 -> Sub1/1
  sfix16_En4/1 -> Sub1/2

== system motor_kit_sim_20MHz/MotorModel/MM_16fixed/MotorElectromagnetics_DSPBA_16fixed/Park_16fixed2 ==
  note: Transformation from Alpha-Beta to dq alignment.
      | Just a rotation, no change in magnitude:
      |
      | xd = xAlpha*cos(Theta_rad) + xBeta*sin(Theta_rad)
      | xq = -xAlpha*sin(Theta_rad) + xBeta*cos(Theta_rad)
  xAlphaBeta : Inport
  cos_phi_el : Inport  Port=2
  sin_phi_el : Inport  Port=3
  Add : DSPBAPrim/Add  primtype=add  nInputs=evalAionMaskParam(gcb,'value',1)  nOutputs=1  omode=Inherit via internal rule with word growth  otype=sfix(17)  scale=constScaleVoltage  rndmethod=Unbiased  factor=1  satmethod=Symmetric  shift_vec=[0 1 2 -1]  value=2  inPortNames=[' '; ' ';]  outPortNames=[' ']  dspbaimage=dspba_prim.svg  text=fprintf('+');  style=Optimised  visibilities=1032  genFPC=off  floatRounding=correct  advOptions=[]  version=20211007
  Demux1 : Demux  Outputs=2
  Mult{1..4} (4 alike) : DSPBAPrim/Mult  primtype=mult  nInputs=2  nOutputs=1  omode=Inherit via internal rule  otype=DataType  scale=constScaleVoltage  rndmethod=Unbiased  factor=1  satmethod=Symmetric  shift_vec=[0 1 2 -1]  value=0  inPortNames=[' '; ' ';]  outPortNames=[' ']  dspbaimage=dspba_prim.svg  text=fprintf('X');  style=Optimised  visibilities=8+2^18+2^19  floatPrecision=float32_m23  floatRounding=correct  advOptions=[]  version=20211007
  Mux1 : Mux  Inputs=2
  Sub1 : DSPBAPrim/Sub  primtype=sub  nInputs=2  nOutputs=1  omode=Inherit via internal rule with word growth  otype=sfix(17)  scale=constScaleVoltage  rndmethod=Unbiased  factor=1  satmethod=Symmetric  shift_vec=[0 1 2 -1]  value=0  inPortNames=['+'; '-';]  outPortNames=[' ']  dspbaimage=dspba_prim.svg  text=fprintf('-');  style=Optimised  visibilities=8  floatRounding=correct  advOptions=[]  version=20211007
  sfix16_{0..5} (6 alike) : DSPBAPrim/Convert  primtype=convert  nInputs=1  nOutputs=1  omode=Specify via dialog  otype=DataType  scale=constScaleVoltage  rndmethod=Unbiased  factor=1  satmethod=Symmetric  shift_vec=[0 1 2 -1]  value=round([0:255]/17)  inPortNames=[' '; ' ';]  outPortNames=[' '; 'c']  dspbaimage=dspba_prim_wide.svg  text=fprintf('convert');  style=Optimised  visibilities=8+64+256+2^17  clipdetect=off  floatPrecision=float32_m23  advOptions=[]  version=20211007
  x_dq : Outport
  wires:
  xAlphaBeta/1 -> Demux1/1
  Mult3/1 -> sfix16_2/1
  Mult4/1 -> sfix16_3/1
  Demux1/1 -> Mult1/1, Mult4/1
  Mult2/1 -> sfix16_1/1
  Mult1/1 -> sfix16_0/1
  Add/1 -> sfix16_4/1
  Sub1/1 -> sfix16_5/1
  Mux1/1 -> x_dq/1
  sin_phi_el/1 -> Mult4/2, Mult2/2
  Demux1/2 -> Mult2/1, Mult3/1
  cos_phi_el/1 -> Mult3/2, Mult1/2
  sfix16_0/1 -> Add/1
  sfix16_1/1 -> Add/2
  sfix16_2/1 -> Sub1/1
  sfix16_3/1 -> Sub1/2
  sfix16_4/1 -> Mux1/1
  sfix16_5/1 -> Mux1/2

== system motor_kit_sim_20MHz/MotorModel/MM_16fixed/MotorElectromagnetics_DSPBA_16fixed/inv_Clarke_16fixed ==
  note: Transformation from equivalent Alpha-Beta 2-phase stator-based values to original 3-phase stator coil values.
      | Scaling chosen so peak values remain the same.
      | Transformation equations:
      |
      | xa = xAlpha
      | xb = -0.5*xAlpha + 0.5*sqrt(3)*xBeta
      | xc = -0.5*xAlpha - 0.5*sqrt(3)*xBeta
  xAlphaBeta : Inport
  Add : DSPBAPrim/Add  primtype=add  nInputs=evalAionMaskParam(gcb,'value',1)  nOutputs=1  omode=Inherit via internal rule with word growth  otype=sfix(17)  scale=constScaleCurrent  rndmethod=Unbiased  factor=1  satmethod=Symmetric  shift_vec=[0 1 2 -1]  value=2  inPortNames=[' '; ' ';]  outPortNames=[' ']  dspbaimage=dspba_prim.svg  text=fprintf('+');  style=Optimised  visibilities=1032+2^17+2^18+2^19  genFPC=off  floatRounding=correct  advOptions=[]  version=20211007
  Demux1 : Demux  Outputs=2
  Mux1 : Mux  Inputs=3
  Sub3 : DSPBAPrim/Sub  primtype=sub  nInputs=2  nOutputs=1  omode=Inherit via internal rule with word growth  otype=sfix(17)  scale=constScaleCurrent  rndmethod=Unbiased  factor=1  satmethod=Symmetric  shift_vec=[0 1 2 -1]  value=0  inPortNames=['+'; '-';]  outPortNames=[' ']  dspbaimage=dspba_prim.svg  text=fprintf('-');  style=Optimised  visibilities=8+2^17+2^18  floatRounding=correct  advOptions=[]  version=20211007
  Subsystem1 : Subsystem  mask{constVal=-1/2}
      mask prompts: constVal "Gain"
      mask Display:
      | color('w');
      | set_param(gcb,'BackgroundColor','yellow');
      | fprintf('Gain\n%s', num2str(constVal));
      | port_label('input',1, 'a');
      | port_label('output',1,'b');
  Subsystem4 : Subsystem  mask{constVal=sqrt(3)}
      mask prompts: constVal "Gain"
      mask Display:
      | color('w');
      | set_param(gcb,'BackgroundColor','yellow');
      | fprintf('sqrt(3)\n', num2str(constVal));
      | port_label('input', 1, 'a');
      | port_label('output', 1, 'b');
  Subsystem5 : Subsystem  mask{constVal=1/2}
      mask prompts: constVal "Gain"
      mask Display:
      | color('w');
      | set_param(gcb,'BackgroundColor','yellow');
      | fprintf('Gain\n%s', num2str(constVal));
      | port_label('input',1, 'a');
      | port_label('output',1,'b');
  sfix16_1 : DSPBAPrim/Convert  primtype=convert  nInputs=1  nOutputs=1  omode=Specify via dialog  otype=DataType  scale=constScaleCurrent  rndmethod=Unbiased  factor=1  satmethod=Symmetric  shift_vec=[0 1 2 -1]  value=round([0:255]/17)  inPortNames=[' '; ' ';]  outPortNames=[' '; 'c']  dspbaimage=dspba_prim_wide.svg  text=fprintf('convert');  style=Optimised  visibilities=8+64+256+2^17  clipdetect=off  floatPrecision=float32_m23  advOptions=[]  version=20211007
  sfix16_2 : DSPBAPrim/Convert  primtype=convert  nInputs=1  nOutputs=1  omode=Specify via dialog  otype=DataType  scale=constScaleCurrent  rndmethod=Unbiased  factor=1  satmethod=Symmetric  shift_vec=[0 1 2 -1]  value=round([0:255]/17)  inPortNames=[' '; ' ';]  outPortNames=[' '; 'c']  dspbaimage=dspba_prim_wide.svg  text=fprintf('convert');  style=Optimised  visibilities=8+64+256+2^17  clipdetect=off  floatPrecision=float32_m23  advOptions=[]  version=20211007
  sfix16_4 : DSPBAPrim/Convert  primtype=convert  nInputs=1  nOutputs=1  omode=Specify via dialog  otype=DataType  scale=constScaleCurrent  rndmethod=Unbiased  factor=1  satmethod=Symmetric  shift_vec=[0 1 2 -1]  value=round([0:255]/17)  inPortNames=[' '; ' ';]  outPortNames=[' '; 'c']  dspbaimage=dspba_prim_wide.svg  text=fprintf('convert');  style=Optimised  visibilities=8+64+256+2^17  clipdetect=off  floatPrecision=float32_m23  advOptions=[]  version=20211007
  xabc : Outport
  wires:
  Subsystem5/1(Out1) -> Subsystem4/1(In1)
  Demux1/2 -> Subsystem5/1(In1)
  Demux1/1 -> sfix16_2/1, Subsystem1/1(In1)  "xa"
  Add/1 -> sfix16_1/1  "xb"
  Mux1/1 -> xabc/1
  Subsystem4/1(Out1) -> Sub3/2, Add/1
  Subsystem1/1(Out1) -> Sub3/1, Add/2
  xAlphaBeta/1 -> Demux1/1
  Sub3/1 -> sfix16_4/1  "xc"
  sfix16_1/1 -> Mux1/2
  sfix16_4/1 -> Mux1/3
  sfix16_2/1 -> Mux1/1

== system motor_kit_sim_20MHz/MotorModel/MM_16fixed/MotorElectromagnetics_DSPBA_16fixed/sine_cosine_16fixed ==
  note: 2 sine blocks are used to calculate sine and cosine.
      | This allows the ALU folder to reduce resource usage.
  pole pairs : Inport
  theta mechanical one turn : Inport  Port=2
  Const : DSPBAPrim/Const  primtype=const  nInputs=0  nOutputs=1  omode=Specify via dialog  otype=ufix(16)  scale=2^-14  rndmethod=Unbiased  factor=1  satmethod=Symmetric  shift_vec=[0 1 2 -1]  value=2  inPortNames=['+'; '+';]  outPortNames=[' ']  dspbaimage=dspba_prim.svg  text=fprintf('%s', num2str(value));  style=Optimised  visibilities=8 + 1024  floatPrecision=float26_m17  warnSaturation=on  version=20211007  SampleTime=inf
  Const1 : DSPBAPrim/Const  primtype=const  nInputs=0  nOutputs=1  omode=Specify via dialog  otype=ufix(16)  scale=2^-14  rndmethod=Unbiased  factor=1  satmethod=Symmetric  shift_vec=[0 1 2 -1]  value=1/2  inPortNames=['+'; '+';]  outPortNames=[' ']  dspbaimage=dspba_prim.svg  text=fprintf('%s', num2str(value));  style=Optimised  visibilities=8 + 1024  floatPrecision=float26_m17  warnSaturation=on  version=20211007  SampleTime=inf
  Mult1 : DSPBAPrim/Mult  primtype=mult  nInputs=2  nOutputs=1  omode=Inherit via internal rule  otype=DataType  scale=2^-14  rndmethod=Unbiased  factor=1  satmethod=Symmetric  shift_vec=[0 1 2 -1]  value=0  inPortNames=[' '; ' ';]  outPortNames=[' ']  dspbaimage=dspba_prim.svg  text=fprintf('X');  style=Optimised  visibilities=8+2^18+2^19  floatPrecision=float32_m23  floatRounding=correct  advOptions=[]  version=20211007
  Mult2 : DSPBAPrim/Mult  primtype=mult  nInputs=2  nOutputs=1  omode=Inherit via internal rule  otype=ufix(16)  scale=2^-14  rndmethod=Unbiased  factor=1  satmethod=Symmetric  shift_vec=[0 1 2 -1]  value=0  inPortNames=[' '; ' ';]  outPortNames=[' ']  dspbaimage=dspba_prim.svg  text=fprintf('X');  style=Optimised  visibilities=8+2^18+2^19  floatPrecision=float32_m23  floatRounding=correct  advOptions=[]  version=20211007
  Sub : DSPBAPrim/Sub  primtype=sub  nInputs=2  nOutputs=1  omode=Inherit via internal rule with word growth  otype=ufix(17)  scale=2^-14  rndmethod=Unbiased  factor=1  satmethod=Symmetric  shift_vec=[0 1 2 -1]  value=0  inPortNames=['+'; '-';]  outPortNames=[' ']  dspbaimage=dspba_prim.svg  text=fprintf('-');  style=Optimised  visibilities=8+2^17+2^18  floatRounding=correct  advOptions=[]  version=20211007
  Trig1 : DSPBAPrim/Trig  primtype=trigfunc  nInputs=1  nOutputs=1  omode=Inherit via internal rule  otype=sfix(16)  scale=2^-15  rndmethod=Unbiased  factor=1  satmethod=Symmetric  shift_vec=[0 1 2 -1]  value=round([0:255]/17)  inPortNames=[' '; ' ';]  outPortNames=[' ']  dspbaimage=dspba_prim_float.svg  text=fprintf('sin(a)');  style=Optimised  visibilities=2^17+2^18  functionExpr=sin(pi*x)  advOptions=[]  version=20211007
  Trig2 : DSPBAPrim/Trig  primtype=trigfunc  nInputs=1  nOutputs=1  omode=Inherit via internal rule  otype=sfix(16)  scale=2^-15  rndmethod=Unbiased  factor=1  satmethod=Symmetric  shift_vec=[0 1 2 -1]  value=round([0:255]/17)  inPortNames=[' '; ' ';]  outPortNames=[' ']  dspbaimage=dspba_prim_float.svg  text=fprintf('sin(a)');  style=Optimised  visibilities=2^17+2^18  functionExpr=sin(pi*x)  advOptions=[]  version=20211007
  modulus : Subsystem
  sfix16_En13_0 : DSPBAPrim/Convert  primtype=convert  nInputs=1  nOutputs=1  omode=Specify via dialog  otype=DataTypeU  scale=constScaleSinCos  rndmethod=Unbiased  factor=1  satmethod=None  shift_vec=[0 1 2 -1]  value=round([0:255]/17)  inPortNames=[' '; ' ';]  outPortNames=[' '; 'c']  dspbaimage=dspba_prim_wide.svg  text=fprintf('convert');  style=Optimised  visibilities=8+64+256+2^17  clipdetect=off  floatPrecision=float32_m23  advOptions=[]  version=20211007
  sfix16_En13_2 : DSPBAPrim/Convert  primtype=convert  nInputs=1  nOutputs=1  omode=Specify via dialog  otype=DataTypeU  scale=constScaleSinCos  rndmethod=Unbiased  factor=1  satmethod=None  shift_vec=[0 1 2 -1]  value=round([0:255]/17)  inPortNames=[' '; ' ';]  outPortNames=[' '; 'c']  dspbaimage=dspba_prim_wide.svg  text=fprintf('convert');  style=Optimised  visibilities=8+64+256+2^17  clipdetect=off  floatPrecision=float32_m23  advOptions=[]  version=20211007
  sfix16_En9 : DSPBAPrim/Convert  primtype=convert  nInputs=1  nOutputs=1  omode=Specify via dialog  otype=DataType  scale=constScaleTrig  rndmethod=Unbiased  factor=1  satmethod=Symmetric  shift_vec=[0 1 2 -1]  value=round([0:255]/17)  inPortNames=[' '; ' ';]  outPortNames=[' '; 'c']  dspbaimage=dspba_prim_wide.svg  text=fprintf('convert');  style=Optimised  visibilities=8+64+256+2^17  clipdetect=off  floatPrecision=float32_m23  advOptions=[]  version=20211007
  sine : Outport
  cosine : Outport  Port=2
  wires:
  modulus/1(Out1) -> Mult2/1
  Mult1/1 -> sfix16_En9/1
  Const/1 -> Mult2/2
  theta mechanical one turn/1 -> Mult1/2
  Const1/1 -> Sub/1
  pole pairs/1 -> Mult1/1
  Trig1/1 -> sine/1
  Mult2/1 -> sfix16_En13_0/1
  sfix16_En9/1 -> modulus/1(In1)
  sfix16_En13_0/1 -> Trig1/1, Sub/2
  Sub/1 -> sfix16_En13_2/1
  Trig2/1 -> cosine/1
  sfix16_En13_2/1 -> Trig2/1

== system motor_kit_sim_20MHz/MotorModel/MM_16fixed/MotorInertia_DSPBA_16fixed/Subsystem3 ==
  In1 : Inport
  Const : DSPBAPrim/Const  primtype=const  nInputs=0  nOutputs=1  omode=Specify via dialog  otype=ufix(16)  scale=2^-18  rndmethod=Unbiased  factor=1  satmethod=Symmetric  shift_vec=[0 1 2 -1]  value=constVal  inPortNames=['+'; '+';]  outPortNames=[' ']  dspbaimage=dspba_prim.svg  text=fprintf('%s', num2str(value));  style=Optimised  visibilities=8 + 1024  floatPrecision=float32_m23  warnSaturation=on  version=20211007  SampleTime=inf
  Mult : DSPBAPrim/Mult  primtype=mult  nInputs=2  nOutputs=1  omode=Inherit via internal rule  otype=sfix(32)  scale=2^-28  rndmethod=Unbiased  factor=1  satmethod=Symmetric  shift_vec=[0 1 2 -1]  value=0  inPortNames=[' '; ' ';]  outPortNames=[' ']  dspbaimage=dspba_prim.svg  text=fprintf('X');  style=Optimised  visibilities=8+2^18+2^19  floatPrecision=float32_m23  floatRounding=correct  advOptions=[]  version=20211007
  Out1 : Outport
  wires:
  Mult/1 -> Out1/1
  In1/1 -> Mult/1
  Const/1 -> Mult/2

== system motor_kit_sim_20MHz/MotorModel/MM_16fixed/MotorElectromagnetics_DSPBA_16fixed/Clarke_16fixed/Subsystem1 ==
  In1 : Inport
  Const3 : DSPBAPrim/Const  primtype=const  nInputs=0  nOutputs=1  omode=Specify via dialog  otype=DataType  scale=2^-15  rndmethod=Unbiased  factor=1  satmethod=Symmetric  shift_vec=[0 1 2 -1]  value=constVal  inPortNames=['+'; '+';]  outPortNames=[' ']  dspbaimage=dspba_prim.svg  text=fprintf('%s', num2str(value));  style=Optimised  visibilities=8 + 1024  floatPrecision=float32_m23  warnSaturation=on  version=20211007  SampleTime=inf
  Mult1 : DSPBAPrim/Mult  primtype=mult  nInputs=2  nOutputs=1  omode=Inherit via internal rule  otype=DataType  scale=constScaleVoltage  rndmethod=Unbiased  factor=1  satmethod=Symmetric  shift_vec=[0 1 2 -1]  value=0  inPortNames=[' '; ' ';]  outPortNames=[' ']  dspbaimage=dspba_prim.svg  text=fprintf('X');  style=Optimised  visibilities=8+2^18+2^19  floatPrecision=float32_m23  floatRounding=correct  advOptions=[]  version=20211007
  Out1 : Outport
  wires:
  In1/1 -> Mult1/1
  Mult1/1 -> Out1/1
  Const3/1 -> Mult1/2

== system motor_kit_sim_20MHz/MotorModel/MM_16fixed/MotorElectromagnetics_DSPBA_16fixed/Clarke_16fixed/Subsystem2 ==
  In1 : Inport
  Const3 : DSPBAPrim/Const  primtype=const  nInputs=0  nOutputs=1  omode=Specify via dialog  otype=DataType  scale=2^-15  rndmethod=Unbiased  factor=1  satmethod=Symmetric  shift_vec=[0 1 2 -1]  value=constVal  inPortNames=['+'; '+';]  outPortNames=[' ']  dspbaimage=dspba_prim.svg  text=fprintf('%s', num2str(value));  style=Optimised  visibilities=8 + 1024  floatPrecision=float32_m23  warnSaturation=on  version=20211007  SampleTime=inf
  Mult1 : DSPBAPrim/Mult  primtype=mult  nInputs=2  nOutputs=1  omode=Inherit via internal rule  otype=DataType  scale=constScaleVoltage  rndmethod=Unbiased  factor=1  satmethod=Symmetric  shift_vec=[0 1 2 -1]  value=0  inPortNames=[' '; ' ';]  outPortNames=[' ']  dspbaimage=dspba_prim.svg  text=fprintf('X');  style=Optimised  visibilities=8+2^18+2^19  floatPrecision=float32_m23  floatRounding=correct  advOptions=[]  version=20211007
  Out1 : Outport
  wires:
  In1/1 -> Mult1/1
  Mult1/1 -> Out1/1
  Const3/1 -> Mult1/2

== system motor_kit_sim_20MHz/MotorModel/MM_16fixed/MotorElectromagnetics_DSPBA_16fixed/Clarke_16fixed/Subsystem6 ==
  In1 : Inport
  Const3 : DSPBAPrim/Const  primtype=const  nInputs=0  nOutputs=1  omode=Specify via dialog  otype=DataType  scale=2^-15  rndmethod=Unbiased  factor=1  satmethod=Symmetric  shift_vec=[0 1 2 -1]  value=constVal  inPortNames=['+'; '+';]  outPortNames=[' ']  dspbaimage=dspba_prim.svg  text=fprintf('%s', num2str(value));  style=Optimised  visibilities=8 + 1024  floatPrecision=float32_m23  warnSaturation=on  version=20211007  SampleTime=inf
  Mult1 : DSPBAPrim/Mult  primtype=mult  nInputs=2  nOutputs=1  omode=Inherit via internal rule  otype=DataType  scale=constScaleVoltage  rndmethod=Unbiased  factor=1  satmethod=Symmetric  shift_vec=[0 1 2 -1]  value=0  inPortNames=[' '; ' ';]  outPortNames=[' ']  dspbaimage=dspba_prim.svg  text=fprintf('X');  style=Optimised  visibilities=8+2^18+2^19  floatPrecision=float32_m23  floatRounding=correct  advOptions=[]  version=20211007
  Out1 : Outport
  wires:
  Const3/1 -> Mult1/2
  Mult1/1 -> Out1/1
  In1/1 -> Mult1/1
